simulink model "PowerSupplyTesting"  (R2022b)
settings: Solver=VariableStepAuto  StartTime=0.0  StopTime=10.0  RelTol=1e-3
libraries: fl_lib x60, ee_lib x28, batteryecm_lib x4
settings Model: Creator=minar  LastModifiedBy=minar

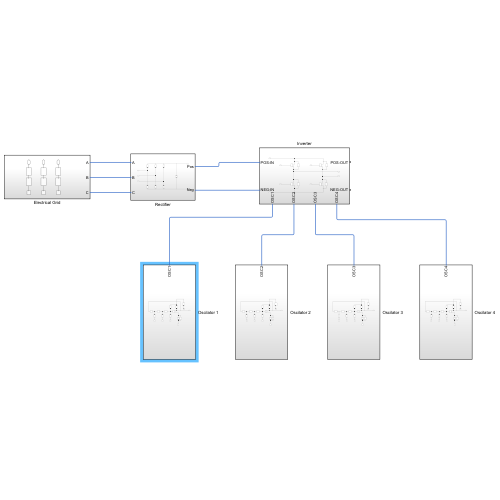
[thumbnail: Simulink's stored preview of the top-level diagram]
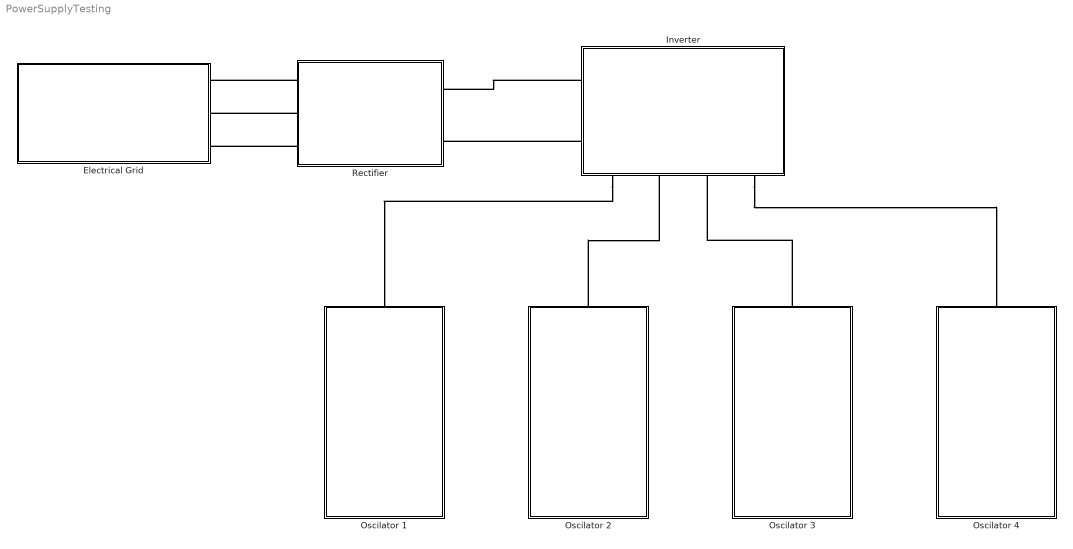
== system PowerSupplyTesting ==
  Electrical Grid : Subsystem
  Inverter : Subsystem
      settings: PortSchema="{\"entries\":[{\"content\":{\"sides\":[{\"content\":{\"connectorIds\":[\"LConn1\",\"LConn2\"]},\"type\":\"ConnectorPlacement.EquallySpacedRectSide\",\"uuid\":\"f7f5b9d2-2f28-4702-8197-1131bf06a0c8\"},{\"content\":{\"connectorIds\":[\"RConn1\",\"RConn2\"],\"side\":\"RIGHT\"},\"type\":\"ConnectorPlacement.EquallySpacedRectSide\",\"uuid\":\"68d9e126-9161-438e-ab0e-3e31da424ef3\"},{\"content\":{\"connectorIds\":[],\"side\":\"TOP\"},\"type\":\"ConnectorPlacement.EquallySpacedRectSide\",\"uuid\":\"a7ff2f77-40f7-4f33-b738-27e4211ddf2a\"},{\"content\":{\"connectorIds\":[\"RConn3\",\"RConn4\",\"RConn5\",\"RConn6\"],\"side\":\"BOTTOM\"},\"type\":\"ConnectorPlacement.EquallySpacedRectSide\",\"uuid\":\"8e7afd57-a60f-4a52-b345-b2d1ae69a6c4\"}]},\"type\":\"ConnectorPlacement.EquallySpacedConnector\",\"uuid\":\"2195a2bc-5e19-43d1-a283-5b386a715552\"}],\"packageUris\":[\"http://schema.mathworks.com/mf0/Connector/R2020b\"],\"version\":\"1.0\"}"
  Oscilator 1 : Subsystem
  Oscilator 2 : Subsystem
  Oscilator 3 : Subsystem
  Oscilator 4 : Subsystem
  Rectifier : Subsystem
  connections:
  Rectifier/RConn1 -- Electrical Grid/RConn1
  Rectifier/RConn2 -- Electrical Grid/RConn2
  Rectifier/RConn3 -- Electrical Grid/RConn3
  Inverter/LConn2 -- Rectifier/LConn2
  Inverter/LConn1 -- Rectifier/LConn1
  Oscilator 3/RConn1 -- Inverter/RConn5
  Oscilator 2/RConn1 -- Inverter/RConn4
  Inverter/RConn3 -- Oscilator 1/RConn1
  Inverter/RConn6 -- Oscilator 4/RConn1

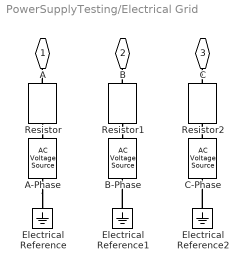
== system PowerSupplyTesting/Electrical Grid ==
  A-Phase : fl_lib/Electrical/Electrical Sources/AC Voltage Source  amp=208 V  shift=0 deg  frequency=60 Hz  omega=0 rad/s
  B-Phase : fl_lib/Electrical/Electrical Sources/AC Voltage Source  amp=208 V  shift=-120 deg  frequency=60 Hz  omega=0 rad/s
  C-Phase : fl_lib/Electrical/Electrical Sources/AC Voltage Source  amp=208 V  shift=-240 deg  frequency=60 Hz  omega=0 rad/s
  Electrical Reference : fl_lib/Electrical/Electrical Elements/Electrical Reference
  Electrical Reference1 : fl_lib/Electrical/Electrical Elements/Electrical Reference
  Electrical Reference2 : fl_lib/Electrical/Electrical Elements/Electrical Reference
  Resistor : fl_lib/Electrical/Electrical Elements/Resistor  R=0.1 Ohm  i_specify=off  i_priority=None  i=0 A  i_nominal_specify=off  i_nominal_unit=A  i_nominal_value=1  v_specify=off  v_priority=None  v=0 V  v_nominal_specify=off  v_nominal_unit=V  v_nominal_value=1
  Resistor1 : fl_lib/Electrical/Electrical Elements/Resistor  R=0.1 Ohm  i_specify=off  i_priority=None  i=0 A  i_nominal_specify=off  i_nominal_unit=A  i_nominal_value=1  v_specify=off  v_priority=None  v=0 V  v_nominal_specify=off  v_nominal_unit=V  v_nominal_value=1
  Resistor2 : fl_lib/Electrical/Electrical Elements/Resistor  R=0.1 Ohm  i_specify=off  i_priority=None  i=0 A  i_nominal_specify=off  i_nominal_unit=A  i_nominal_value=1  v_specify=off  v_priority=None  v=0 V  v_nominal_specify=off  v_nominal_unit=V  v_nominal_value=1
  A : PMIOPort  Side=Right
  B : PMIOPort  Port=2  Side=Right
  C : PMIOPort  Port=3  Side=Right
  connections:
  C-Phase/LConn1 -- Resistor2/RConn1
  A-Phase/RConn1 -- Electrical Reference/LConn1
  Electrical Reference1/LConn1 -- B-Phase/RConn1
  Electrical Reference2/LConn1 -- C-Phase/RConn1
  Resistor/LConn1 -- A/RConn1
  Resistor/RConn1 -- A-Phase/LConn1
  Resistor1/LConn1 -- B/RConn1
  Resistor1/RConn1 -- B-Phase/LConn1
  Resistor2/LConn1 -- C/RConn1

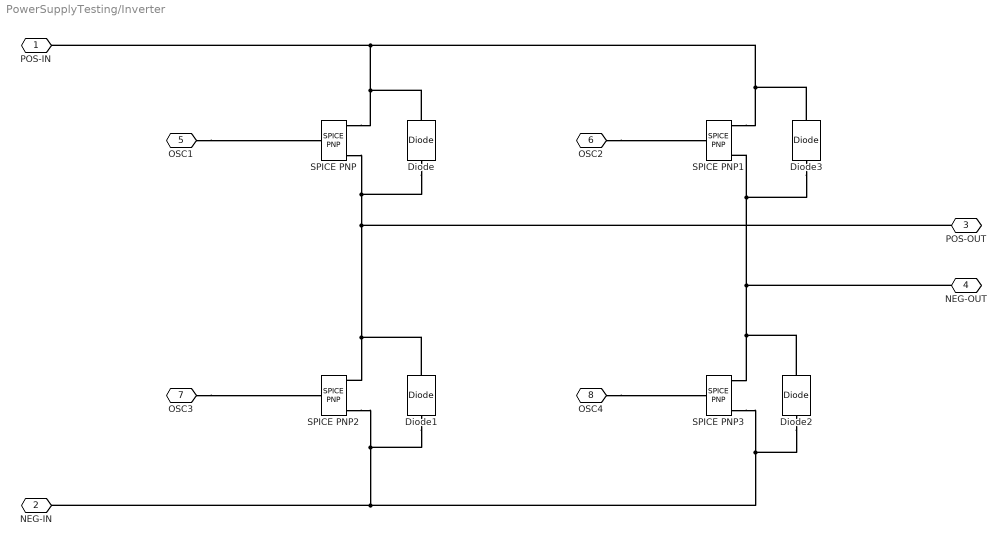
== system PowerSupplyTesting/Inverter ==
  Diode{,1..3} (4 alike) : ee_lib/Semiconductors & Converters/Diode  ModelType=ee.enum.diode.modelType.pwl  TableType=ee.enum.diode.tableType.IfMat  IfMat=[.07, .12, .19, 1.75, 4.24, 7.32, 11.2; .16, .3, .72, 2.14, 5.02, 8.35, 13.12] A  VfMat=[.9, 1.15, 1.25, 1.5, 1.75, 2.17, 2.6, 2.85; .58, .68, .75, 1.1, 1.38, 1.77, 2.27, 2.7] V  TjVec=[25, 125] degC  VfVec=[.5, .7, .9, 1.3, 1.7, 2.1, 2.5] V  IfVec=[.1, .2, .5, 1, 2, 4, 7, 10] A  Vf=0.6 V  Ron=0.3 Ohm  Goff=1e-8 S  prmExp=ee.enum.diode.expParam.useTwo  I12=[.0137, .545] A  V12=[.6, .7] V  RS=0 Ohm  Tmeas=25 degC  IS=1e-12 A  ec=1  I1=0.0137 A  V1=0.6 V  N_series=1  N_parallel=1  Rz=0.3 Ohm  BV=inf V  C_param=ee.enum.diode.capParam.fixed  CJ=0 pF  CJ0=5 pF  Vvec=[.1, 10, 100] V  Cvec=[3.5, 1, .4] pF  VJ=1 V  Mgrad=0.5  FC=0.5  Q_param=ee.enum.diode.recoveryParam.off  iRM=-7.15 A  iF=4 A  didt=-750 A/us  trr_factor=3  trr=115 ns  Qrr=150 nA*s  Vr=-600 V  Ls=150 nH  Erec=0.03 J  TT=50 ns  tau=100 ns  T_param=ee.enum.diode.temperatureParam.off  Tdevice=25 degC  I1_T2=0.245 A  V1_T2=0.5 V  IS_T2=1.25e-7 A  Tmeas2=125 degC  XTI_param=ee.enum.diode.xtiParam.pn  XTI=3  EG_param=ee.enum.diode.egapParam.material_si  EG=1.11 eV  dBVdT=0 V/K  enable_faults=simscape.enum.onoff.off  fault_action=simscape.enum.assert.action.none  fault_types=ee.enum.diode.faults.open  tau_fault=1e-3 s  IfMat_faulted=[.07, .12, .19, 1.75, 4.24, 7.32, 11.2; .16, .3, .72, 2.14, 4.02, 6.35, 9.12] A  VfMat_faulted=[.9, 1.15, 1.25, 1.5, 1.75, 2.17, 2.6, 2.85; .58, .68, .75, 1.1, 1.38, 1.77, 2.27, 2.7] V  VfVec_faulted=[.5, .7, .9, 1.3, 1.7, 2.1, 2.5] V  IfVec_faulted=[.1, .2, .5, 1, 2, 4, 7, 10] A  Ropen_faulted=1000 Ohm  Gshort_faulted=1000 1/Ohm  Vf_faulted=0.6 V  Ron_faulted=0.3 Ohm  Goff_faulted=1e-8 S  I12_faulted=[.0137, .545] A  V12_faulted=[.6, .7] V  IS_faulted=1e-12 A  ec_faulted=1  I1_faulted=0.0137 A  V1_faulted=0.6 V  RS_faulted=0 Ohm  Rz_faulted=0.3 Ohm  BV_faulted=inf V  Cscale_faulted=100  enable_temporal_fault=simscape.enum.onoff.off  t_fault=inf s  enable_behavioral_fault=simscape.enum.onoff.off  max_permissible_voltage=inf V  n_fail_on_voltage=1  max_permissible_current=inf A  t_fail_on_current=1 s  max_permissible_dVdt=inf V/s  enable_fault_input=simscape.enum.onoff.off  i_specify=off  i_priority=None  i=0 A  i_nominal_specify=off  i_nominal_unit=A  i_nominal_value=1  v_specify=off  v_priority=None  v=0 V  v_nominal_specify=off  v_nominal_unit=V  v_nominal_value=1  v_capacitor_specify=off  v_capacitor_priority=None  v_capacitor=0 V  v_capacitor_nominal_specify=off  v_capacitor_nominal_unit=V  v_capacitor_nominal_value=1  i_diode_specify=off  i_diode_priority=None  i_diode=0 A  i_diode_nominal_specify=off  i_diode_nominal_unit=A  i_diode_nominal_value=1  v_diode_specify=off  v_diode_priority=None  v_diode=0 V  v_diode_nominal_specify=off  v_diode_nominal_unit=V  v_diode_nominal_value=1  i_capacitor_specify=off  i_capacitor_priority=None  i_capacitor=0 A  i_capacitor_nominal_specify=off  i_capacitor_nominal_unit=A  i_capacitor_nominal_value=1  power_dissipated_specify=off  power_dissipated_priority=None  power_dissipated=0 W  power_dissipated_nominal_specify=off  power_dissipated_nominal_unit=W  power_dissipated_nominal_value=1  fidelity_level=ee.enum.diode.fidelity.includeChargeDyn  rec_loss_model=ee.enum.diode.reverseRecoveryModel.fixed  ErecVal=0 J  ErecMat=zeros(2, 3) J  TjrecVec=[298.15, 398.15] K  IfrecVec=[.1, 1, 10] A  VrecVal=10 V  tFilter=1 / 1000 / 100 s  max_permissible_temperature=inf K  t_fail_on_temperature=1 s  thermal_network_parameterization=ee.enum.thermalNetworkTopology.junctionCase  Rth=[0, 10] K/W  Rth_Cauer=[1, 3, 10] K/W  Rth_Foster=[4, 6] K/W  thermal_mass_parameterization=ee.enum.thermalNetwork.timeconstant  thermal_mass=[0, 1] J/K  thermal_mass_Cauer=[.1, .3, 1] J/K  thermal_mass_Foster=[1.5, 3] J/K  thermal_time_constant=[0, 10] s  thermal_time_constant_Cauer=[1, 3, 10] s  thermal_time_constant_Foster=[6, 18] s  thermal_mass_initial_temperatures=[25, 25] degC  thermal_mass_initial_temperatures_Cauer=[25, 25, 25] degC  junction_thermal_mass=0.01 J/K  Tvec_initial_Foster=[25, 25, 25, 25] degC  no_thermal_network=0  junction_temperature_specify=off  junction_temperature_priority=None  junction_temperature=25 degC  junction_temperature_nominal_specify=off  junction_temperature_nominal_unit=degC  junction_temperature_nominal_value=1
  SPICE PNP{,1..3} (4 alike) : ee_lib/Additional Components/SPICE Semiconductors/SPICE PNP  AREA=1.0 m^2  SCALE=1  IS=1.0e-16 A/m^2  BF=100.0  NF=1  VAF=Inf V  IKF=Inf A/m^2  ISE=0 A/m^2  NE=1.5  BR=1  NR=1  VAR=Inf V  IKR=Inf A/m^2  ISC=0 A/m^2  NC=2  RB=1 Ohm*m^2  IRB=Inf A/m^2  RBM=0 Ohm*m^2  RE=1e-4 Ohm*m^2  RC=0.01 Ohm*m^2  C_param=1  FC=0.5  IC_given=1  ICVBE=0 V  ICVCE=0 V  CJE=0 F/m^2  VJE=0.75 V  MJE=0.33  TF=0 s  XTF=0  VTF=Inf V  ITF=0 A/m^2  CJC=0 F/m^2  VJC=0.75 V  MJC=0.33  XCJC=1  TR=0 s  CJS=0 F/m^2  VJS=0.75 V  MJS=0  T_param=1  XTB=0  EG=1.11 eV  XTI=3  TFIXED=300.15 K  TMEAS=300.15 K  TOFFSET=0 K
      settings: InternalSimscapePortConfiguration="{\"Bottom\":[],\"Left\":[{\"id\":\"bx\",\"label\":\"\",\"type\":\"foundation.electrical.electrical\"}],\"Right\":[{\"id\":\"cx\",\"label\":\"\",\"type\":\"foundation.electrical.electrical\"},{\"id\":\"sx\",\"label\":\"s\",\"type\":\"foundation.electrical.electrical\"},{\"id\":\"ex\",\"label\":\"\",\"type\":\"foundation.electrical.electrical\"}],\"Top\":[]}"
  POS-IN : PMIOPort  Side=Left
  NEG-IN : PMIOPort  Port=2  Side=Left
  POS-OUT : PMIOPort  Port=3  Side=Right
  NEG-OUT : PMIOPort  Port=4  Side=Right
  OSC1 : PMIOPort  Port=5  Side=Right
  OSC2 : PMIOPort  Port=6  Side=Right
  OSC3 : PMIOPort  Port=7  Side=Right
  OSC4 : PMIOPort  Port=8  Side=Right
  connections:
  SPICE PNP3/RConn1 -- Diode2/LConn1 -- NEG-OUT/RConn1 -- Diode3/RConn1 -- SPICE PNP1/RConn3
  SPICE PNP/RConn3 -- Diode/RConn1 -- POS-OUT/RConn1 -- Diode1/LConn1 -- SPICE PNP2/RConn1
  OSC1/RConn1 -- SPICE PNP/LConn1
  OSC2/RConn1 -- SPICE PNP1/LConn1
  OSC3/RConn1 -- SPICE PNP2/LConn1
  OSC4/RConn1 -- SPICE PNP3/LConn1
  SPICE PNP2/RConn3 -- Diode1/RConn1 -- Diode2/RConn1 -- SPICE PNP3/RConn3 -- NEG-IN/RConn1
  SPICE PNP/RConn1 -- Diode/LConn1 -- Diode3/LConn1 -- SPICE PNP1/RConn1 -- POS-IN/RConn1

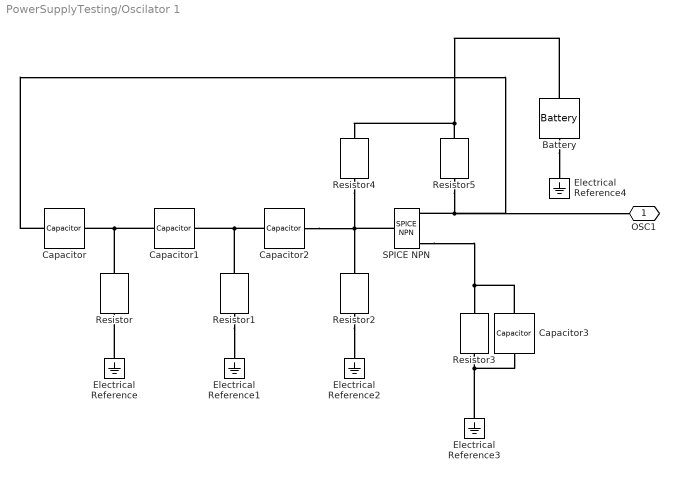
== system PowerSupplyTesting/Oscilator 1 ==
  Battery : batteryecm_lib/Battery  Vnom=12 V  prm_dir=simscape.enum.battery.prm_dir.disabled  R1_dis=2 Ohm  R1_ch=2 Ohm  R1=2 Ohm  prm_AH=simscape.enum.battery.prm_AH.infinite  AH=50 A*hr  V1=11.5 V  AH1=25 A*hr  prm_R2=simscape.enum.battery.prm_R2.disabled  R2=2000 Ohm  prm_dyn=simscape.enum.battery.prm_dyn.off  Rp1=0.005 Ohm  tau1=30 s  Rp2=0.005 Ohm  tau2=30 s  Rp3=0.005 Ohm  tau3=30 s  Rp4=0.005 Ohm  tau4=30 s  Rp5=0.005 Ohm  tau5=30 s  prm_fade=simscape.enum.battery.prm_fade.disabled  N_fade=100  AH_fade=45 A*hr  R1_fade=2.02 Ohm  R1_ch_fade=2.02 Ohm  V1_fade=10.35 V  prm_age=simscape.enum.battery.prm_age.disabled  prm_age_OCV=simscape.enum.battery.prm_age_OCV.OCV  OCV_age=0.9  SOC_age=60  delta_time_age_vec=[0] d  temperature_age_vec=[273] K  OCV_scaling_age=2.2134e6  OCV_offset_age=1.632e6  temp_exp_age=0.515833569 V  t_exp_age=0.75  i_specify=off  i_priority=None  i=0 A  i_nominal_specify=off  i_nominal_unit=A  i_nominal_value=1  v_specify=off  v_priority=None  v=0 V  v_nominal_specify=off  v_nominal_unit=V  v_nominal_value=1  charge_specify=off  charge_priority=High  charge=50 A*hr  charge_nominal_specify=off  charge_nominal_unit=A*hr  charge_nominal_value=1  num_cycles_specify=off  num_cycles_priority=High  num_cycles=0  num_cycles_nominal_specify=off  num_cycles_nominal_unit=1  num_cycles_nominal_value=1  Tmeas=298.15 K  Tmeas_age=298.15 K  Vnom_T2=12 V  R1_T2=2.2 Ohm  R1_T2_dis=2.2 Ohm  R1_T2_ch=2.2 Ohm  V1_T2=11.4 V  R2_T2=2200 Ohm  Rp1_T2=0.005 Ohm  tau1_T2=30 s  Rp2_T2=0.005 Ohm  tau2_T2=30 s  Rp3_T2=0.005 Ohm  tau3_T2=30 s  Rp4_T2=0.005 Ohm  tau4_T2=30 s  Rp5_T2=0.005 Ohm  tau5_T2=30 s  Tmeas2=273.15 K  thermal_mass=30000 J/K  temperature_specify=off  temperature_priority=High  temperature=298.15 K  temperature_nominal_specify=off  temperature_nominal_unit=K  temperature_nominal_value=1
  Capacitor{,1..3} (4 alike) : ee_lib/Passive/Capacitor  cap_option=0  c=1e-6 F  Cvec=[1e-05, 1e-06] F  Vvec=[0, 10] V  CV_table_symmetry=1  f_vec=[1, 10] kHz  DFext_vec=[.8, 1.2]  enable_C_tol=0  C_tol=5  tol_distribution=1  nSigma=4  r=1e-6 Ohm  g=0 1/Ohm  averaging_period=0 s  enable_operating_limits=0  operating_limit_action=2  max_working_voltage_range=[-25, 25] V  power_rating=1 W  enable_faults=0  fault_action=1  Cscale_faulted=100  R_faulted=1e-3 Ohm  G_faulted=0 1/Ohm  tau_fault=1e-3 s  enable_temporal_fault=0  t_fault=1 s  enable_behavioral_fault=0  max_permissible_voltage_range=[-100, 100] V  t_fail_on_voltage=1 s  i_specify=off  i_priority=None  i=0 A  i_nominal_specify=off  i_nominal_unit=A  i_nominal_value=1  v_specify=off  v_priority=None  v=0 V  v_nominal_specify=off  v_nominal_unit=V  v_nominal_value=1  vc_specify=off  vc_priority=High  vc=0 V  vc_nominal_specify=off  vc_nominal_unit=V  vc_nominal_value=1
  Electrical Reference{,1..4} (5 alike) : fl_lib/Electrical/Electrical Elements/Electrical Reference
  Resistor{,1..5} (6 alike) : fl_lib/Electrical/Electrical Elements/Resistor  R=1 Ohm  i_specify=off  i_priority=None  i=0 A  i_nominal_specify=off  i_nominal_unit=A  i_nominal_value=1  v_specify=off  v_priority=None  v=0 V  v_nominal_specify=off  v_nominal_unit=V  v_nominal_value=1
  SPICE NPN : ee_lib/Additional Components/SPICE Semiconductors/SPICE NPN  AREA=1.0 m^2  SCALE=1  IS=1.0e-16 A/m^2  BF=100.0  NF=1  VAF=Inf V  IKF=Inf A/m^2  ISE=0 A/m^2  NE=1.5  BR=1  NR=1  VAR=Inf V  IKR=Inf A/m^2  ISC=0 A/m^2  NC=2  RB=1 Ohm*m^2  IRB=Inf A/m^2  RBM=0 Ohm*m^2  RE=1e-4 Ohm*m^2  RC=0.01 Ohm*m^2  C_param=1  FC=0.5  IC_given=1  ICVBE=0 V  ICVCE=0 V  CJE=0 F/m^2  VJE=0.75 V  MJE=0.33  TF=0 s  XTF=0  VTF=Inf V  ITF=0 A/m^2  CJC=0 F/m^2  VJC=0.75 V  MJC=0.33  XCJC=1  TR=0 s  CJS=0 F/m^2  VJS=0.75 V  MJS=0  T_param=1  XTB=0  EG=1.11 eV  XTI=3  TFIXED=300.15 K  TMEAS=300.15 K  TOFFSET=0 K
      settings: InternalSimscapePortConfiguration="{\"Bottom\":[],\"Left\":[{\"id\":\"bx\",\"label\":\"\",\"type\":\"foundation.electrical.electrical\"}],\"Right\":[{\"id\":\"cx\",\"label\":\"\",\"type\":\"foundation.electrical.electrical\"},{\"id\":\"sx\",\"label\":\"s\",\"type\":\"foundation.electrical.electrical\"},{\"id\":\"ex\",\"label\":\"\",\"type\":\"foundation.electrical.electrical\"}],\"Top\":[]}"
  OSC1 : PMIOPort  Side=Right
  connections:
  SPICE NPN/RConn3 -- Capacitor3/LConn1 -- Resistor3/LConn1
  Capacitor3/RConn1 -- Electrical Reference3/LConn1 -- Resistor3/RConn1
  Resistor5/RConn1 -- OSC1/RConn1 -- Capacitor/LConn1 -- SPICE NPN/RConn1
  Resistor5/LConn1 -- Battery/LConn1 -- Resistor4/LConn1
  Resistor4/RConn1 -- Resistor2/LConn1 -- Capacitor2/RConn1 -- SPICE NPN/LConn1
  Capacitor2/LConn1 -- Capacitor1/RConn1 -- Resistor1/LConn1
  Capacitor1/LConn1 -- Resistor/LConn1 -- Capacitor/RConn1
  Electrical Reference/LConn1 -- Resistor/RConn1
  Resistor1/RConn1 -- Electrical Reference1/LConn1
  Resistor2/RConn1 -- Electrical Reference2/LConn1
  Battery/RConn1 -- Electrical Reference4/LConn1

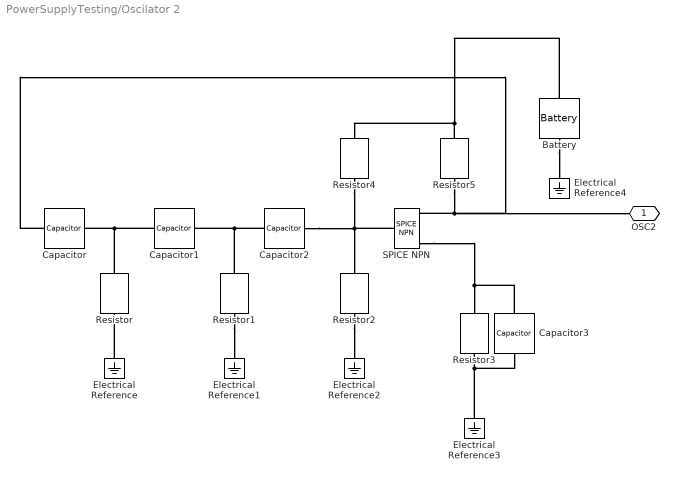
== system PowerSupplyTesting/Oscilator 2 ==
  Battery : batteryecm_lib/Battery  Vnom=12 V  prm_dir=simscape.enum.battery.prm_dir.disabled  R1_dis=2 Ohm  R1_ch=2 Ohm  R1=2 Ohm  prm_AH=simscape.enum.battery.prm_AH.infinite  AH=50 A*hr  V1=11.5 V  AH1=25 A*hr  prm_R2=simscape.enum.battery.prm_R2.disabled  R2=2000 Ohm  prm_dyn=simscape.enum.battery.prm_dyn.off  Rp1=0.005 Ohm  tau1=30 s  Rp2=0.005 Ohm  tau2=30 s  Rp3=0.005 Ohm  tau3=30 s  Rp4=0.005 Ohm  tau4=30 s  Rp5=0.005 Ohm  tau5=30 s  prm_fade=simscape.enum.battery.prm_fade.disabled  N_fade=100  AH_fade=45 A*hr  R1_fade=2.02 Ohm  R1_ch_fade=2.02 Ohm  V1_fade=10.35 V  prm_age=simscape.enum.battery.prm_age.disabled  prm_age_OCV=simscape.enum.battery.prm_age_OCV.OCV  OCV_age=0.9  SOC_age=60  delta_time_age_vec=[0] d  temperature_age_vec=[273] K  OCV_scaling_age=2.2134e6  OCV_offset_age=1.632e6  temp_exp_age=0.515833569 V  t_exp_age=0.75  i_specify=off  i_priority=None  i=0 A  i_nominal_specify=off  i_nominal_unit=A  i_nominal_value=1  v_specify=off  v_priority=None  v=0 V  v_nominal_specify=off  v_nominal_unit=V  v_nominal_value=1  charge_specify=off  charge_priority=High  charge=50 A*hr  charge_nominal_specify=off  charge_nominal_unit=A*hr  charge_nominal_value=1  num_cycles_specify=off  num_cycles_priority=High  num_cycles=0  num_cycles_nominal_specify=off  num_cycles_nominal_unit=1  num_cycles_nominal_value=1  Tmeas=298.15 K  Tmeas_age=298.15 K  Vnom_T2=12 V  R1_T2=2.2 Ohm  R1_T2_dis=2.2 Ohm  R1_T2_ch=2.2 Ohm  V1_T2=11.4 V  R2_T2=2200 Ohm  Rp1_T2=0.005 Ohm  tau1_T2=30 s  Rp2_T2=0.005 Ohm  tau2_T2=30 s  Rp3_T2=0.005 Ohm  tau3_T2=30 s  Rp4_T2=0.005 Ohm  tau4_T2=30 s  Rp5_T2=0.005 Ohm  tau5_T2=30 s  Tmeas2=273.15 K  thermal_mass=30000 J/K  temperature_specify=off  temperature_priority=High  temperature=298.15 K  temperature_nominal_specify=off  temperature_nominal_unit=K  temperature_nominal_value=1
  Capacitor{,1..3} (4 alike) : ee_lib/Passive/Capacitor  cap_option=0  c=1e-6 F  Cvec=[1e-05, 1e-06] F  Vvec=[0, 10] V  CV_table_symmetry=1  f_vec=[1, 10] kHz  DFext_vec=[.8, 1.2]  enable_C_tol=0  C_tol=5  tol_distribution=1  nSigma=4  r=1e-6 Ohm  g=0 1/Ohm  averaging_period=0 s  enable_operating_limits=0  operating_limit_action=2  max_working_voltage_range=[-25, 25] V  power_rating=1 W  enable_faults=0  fault_action=1  Cscale_faulted=100  R_faulted=1e-3 Ohm  G_faulted=0 1/Ohm  tau_fault=1e-3 s  enable_temporal_fault=0  t_fault=1 s  enable_behavioral_fault=0  max_permissible_voltage_range=[-100, 100] V  t_fail_on_voltage=1 s  i_specify=off  i_priority=None  i=0 A  i_nominal_specify=off  i_nominal_unit=A  i_nominal_value=1  v_specify=off  v_priority=None  v=0 V  v_nominal_specify=off  v_nominal_unit=V  v_nominal_value=1  vc_specify=off  vc_priority=High  vc=0 V  vc_nominal_specify=off  vc_nominal_unit=V  vc_nominal_value=1
  Electrical Reference{,1..4} (5 alike) : fl_lib/Electrical/Electrical Elements/Electrical Reference
  Resistor{,1..5} (6 alike) : fl_lib/Electrical/Electrical Elements/Resistor  R=1 Ohm  i_specify=off  i_priority=None  i=0 A  i_nominal_specify=off  i_nominal_unit=A  i_nominal_value=1  v_specify=off  v_priority=None  v=0 V  v_nominal_specify=off  v_nominal_unit=V  v_nominal_value=1
  SPICE NPN : ee_lib/Additional Components/SPICE Semiconductors/SPICE NPN  AREA=1.0 m^2  SCALE=1  IS=1.0e-16 A/m^2  BF=100.0  NF=1  VAF=Inf V  IKF=Inf A/m^2  ISE=0 A/m^2  NE=1.5  BR=1  NR=1  VAR=Inf V  IKR=Inf A/m^2  ISC=0 A/m^2  NC=2  RB=1 Ohm*m^2  IRB=Inf A/m^2  RBM=0 Ohm*m^2  RE=1e-4 Ohm*m^2  RC=0.01 Ohm*m^2  C_param=1  FC=0.5  IC_given=1  ICVBE=0 V  ICVCE=0 V  CJE=0 F/m^2  VJE=0.75 V  MJE=0.33  TF=0 s  XTF=0  VTF=Inf V  ITF=0 A/m^2  CJC=0 F/m^2  VJC=0.75 V  MJC=0.33  XCJC=1  TR=0 s  CJS=0 F/m^2  VJS=0.75 V  MJS=0  T_param=1  XTB=0  EG=1.11 eV  XTI=3  TFIXED=300.15 K  TMEAS=300.15 K  TOFFSET=0 K
      settings: InternalSimscapePortConfiguration="{\"Bottom\":[],\"Left\":[{\"id\":\"bx\",\"label\":\"\",\"type\":\"foundation.electrical.electrical\"}],\"Right\":[{\"id\":\"cx\",\"label\":\"\",\"type\":\"foundation.electrical.electrical\"},{\"id\":\"sx\",\"label\":\"s\",\"type\":\"foundation.electrical.electrical\"},{\"id\":\"ex\",\"label\":\"\",\"type\":\"foundation.electrical.electrical\"}],\"Top\":[]}"
  OSC2 : PMIOPort  Side=Right
  connections:
  SPICE NPN/RConn3 -- Capacitor3/LConn1 -- Resistor3/LConn1
  Capacitor3/RConn1 -- Electrical Reference3/LConn1 -- Resistor3/RConn1
  Resistor5/RConn1 -- OSC2/RConn1 -- Capacitor/LConn1 -- SPICE NPN/RConn1
  Resistor5/LConn1 -- Battery/LConn1 -- Resistor4/LConn1
  Resistor4/RConn1 -- Resistor2/LConn1 -- Capacitor2/RConn1 -- SPICE NPN/LConn1
  Capacitor2/LConn1 -- Capacitor1/RConn1 -- Resistor1/LConn1
  Capacitor1/LConn1 -- Resistor/LConn1 -- Capacitor/RConn1
  Electrical Reference/LConn1 -- Resistor/RConn1
  Resistor1/RConn1 -- Electrical Reference1/LConn1
  Resistor2/RConn1 -- Electrical Reference2/LConn1
  Battery/RConn1 -- Electrical Reference4/LConn1

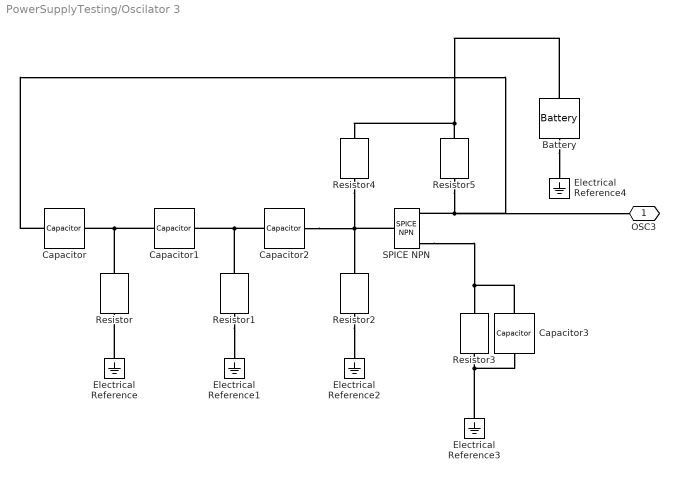
== system PowerSupplyTesting/Oscilator 3 ==
  Battery : batteryecm_lib/Battery  Vnom=12 V  prm_dir=simscape.enum.battery.prm_dir.disabled  R1_dis=2 Ohm  R1_ch=2 Ohm  R1=2 Ohm  prm_AH=simscape.enum.battery.prm_AH.infinite  AH=50 A*hr  V1=11.5 V  AH1=25 A*hr  prm_R2=simscape.enum.battery.prm_R2.disabled  R2=2000 Ohm  prm_dyn=simscape.enum.battery.prm_dyn.off  Rp1=0.005 Ohm  tau1=30 s  Rp2=0.005 Ohm  tau2=30 s  Rp3=0.005 Ohm  tau3=30 s  Rp4=0.005 Ohm  tau4=30 s  Rp5=0.005 Ohm  tau5=30 s  prm_fade=simscape.enum.battery.prm_fade.disabled  N_fade=100  AH_fade=45 A*hr  R1_fade=2.02 Ohm  R1_ch_fade=2.02 Ohm  V1_fade=10.35 V  prm_age=simscape.enum.battery.prm_age.disabled  prm_age_OCV=simscape.enum.battery.prm_age_OCV.OCV  OCV_age=0.9  SOC_age=60  delta_time_age_vec=[0] d  temperature_age_vec=[273] K  OCV_scaling_age=2.2134e6  OCV_offset_age=1.632e6  temp_exp_age=0.515833569 V  t_exp_age=0.75  i_specify=off  i_priority=None  i=0 A  i_nominal_specify=off  i_nominal_unit=A  i_nominal_value=1  v_specify=off  v_priority=None  v=0 V  v_nominal_specify=off  v_nominal_unit=V  v_nominal_value=1  charge_specify=off  charge_priority=High  charge=50 A*hr  charge_nominal_specify=off  charge_nominal_unit=A*hr  charge_nominal_value=1  num_cycles_specify=off  num_cycles_priority=High  num_cycles=0  num_cycles_nominal_specify=off  num_cycles_nominal_unit=1  num_cycles_nominal_value=1  Tmeas=298.15 K  Tmeas_age=298.15 K  Vnom_T2=12 V  R1_T2=2.2 Ohm  R1_T2_dis=2.2 Ohm  R1_T2_ch=2.2 Ohm  V1_T2=11.4 V  R2_T2=2200 Ohm  Rp1_T2=0.005 Ohm  tau1_T2=30 s  Rp2_T2=0.005 Ohm  tau2_T2=30 s  Rp3_T2=0.005 Ohm  tau3_T2=30 s  Rp4_T2=0.005 Ohm  tau4_T2=30 s  Rp5_T2=0.005 Ohm  tau5_T2=30 s  Tmeas2=273.15 K  thermal_mass=30000 J/K  temperature_specify=off  temperature_priority=High  temperature=298.15 K  temperature_nominal_specify=off  temperature_nominal_unit=K  temperature_nominal_value=1
  Capacitor{,1..3} (4 alike) : ee_lib/Passive/Capacitor  cap_option=0  c=1e-6 F  Cvec=[1e-05, 1e-06] F  Vvec=[0, 10] V  CV_table_symmetry=1  f_vec=[1, 10] kHz  DFext_vec=[.8, 1.2]  enable_C_tol=0  C_tol=5  tol_distribution=1  nSigma=4  r=1e-6 Ohm  g=0 1/Ohm  averaging_period=0 s  enable_operating_limits=0  operating_limit_action=2  max_working_voltage_range=[-25, 25] V  power_rating=1 W  enable_faults=0  fault_action=1  Cscale_faulted=100  R_faulted=1e-3 Ohm  G_faulted=0 1/Ohm  tau_fault=1e-3 s  enable_temporal_fault=0  t_fault=1 s  enable_behavioral_fault=0  max_permissible_voltage_range=[-100, 100] V  t_fail_on_voltage=1 s  i_specify=off  i_priority=None  i=0 A  i_nominal_specify=off  i_nominal_unit=A  i_nominal_value=1  v_specify=off  v_priority=None  v=0 V  v_nominal_specify=off  v_nominal_unit=V  v_nominal_value=1  vc_specify=off  vc_priority=High  vc=0 V  vc_nominal_specify=off  vc_nominal_unit=V  vc_nominal_value=1
  Electrical Reference{,1..4} (5 alike) : fl_lib/Electrical/Electrical Elements/Electrical Reference
  Resistor{,1..5} (6 alike) : fl_lib/Electrical/Electrical Elements/Resistor  R=1 Ohm  i_specify=off  i_priority=None  i=0 A  i_nominal_specify=off  i_nominal_unit=A  i_nominal_value=1  v_specify=off  v_priority=None  v=0 V  v_nominal_specify=off  v_nominal_unit=V  v_nominal_value=1
  SPICE NPN : ee_lib/Additional Components/SPICE Semiconductors/SPICE NPN  AREA=1.0 m^2  SCALE=1  IS=1.0e-16 A/m^2  BF=100.0  NF=1  VAF=Inf V  IKF=Inf A/m^2  ISE=0 A/m^2  NE=1.5  BR=1  NR=1  VAR=Inf V  IKR=Inf A/m^2  ISC=0 A/m^2  NC=2  RB=1 Ohm*m^2  IRB=Inf A/m^2  RBM=0 Ohm*m^2  RE=1e-4 Ohm*m^2  RC=0.01 Ohm*m^2  C_param=1  FC=0.5  IC_given=1  ICVBE=0 V  ICVCE=0 V  CJE=0 F/m^2  VJE=0.75 V  MJE=0.33  TF=0 s  XTF=0  VTF=Inf V  ITF=0 A/m^2  CJC=0 F/m^2  VJC=0.75 V  MJC=0.33  XCJC=1  TR=0 s  CJS=0 F/m^2  VJS=0.75 V  MJS=0  T_param=1  XTB=0  EG=1.11 eV  XTI=3  TFIXED=300.15 K  TMEAS=300.15 K  TOFFSET=0 K
      settings: InternalSimscapePortConfiguration="{\"Bottom\":[],\"Left\":[{\"id\":\"bx\",\"label\":\"\",\"type\":\"foundation.electrical.electrical\"}],\"Right\":[{\"id\":\"cx\",\"label\":\"\",\"type\":\"foundation.electrical.electrical\"},{\"id\":\"sx\",\"label\":\"s\",\"type\":\"foundation.electrical.electrical\"},{\"id\":\"ex\",\"label\":\"\",\"type\":\"foundation.electrical.electrical\"}],\"Top\":[]}"
  OSC3 : PMIOPort  Side=Right
  connections:
  SPICE NPN/RConn3 -- Capacitor3/LConn1 -- Resistor3/LConn1
  Capacitor3/RConn1 -- Electrical Reference3/LConn1 -- Resistor3/RConn1
  Resistor5/RConn1 -- OSC3/RConn1 -- Capacitor/LConn1 -- SPICE NPN/RConn1
  Resistor5/LConn1 -- Battery/LConn1 -- Resistor4/LConn1
  Resistor4/RConn1 -- Resistor2/LConn1 -- Capacitor2/RConn1 -- SPICE NPN/LConn1
  Capacitor2/LConn1 -- Capacitor1/RConn1 -- Resistor1/LConn1
  Capacitor1/LConn1 -- Resistor/LConn1 -- Capacitor/RConn1
  Electrical Reference/LConn1 -- Resistor/RConn1
  Resistor1/RConn1 -- Electrical Reference1/LConn1
  Resistor2/RConn1 -- Electrical Reference2/LConn1
  Battery/RConn1 -- Electrical Reference4/LConn1

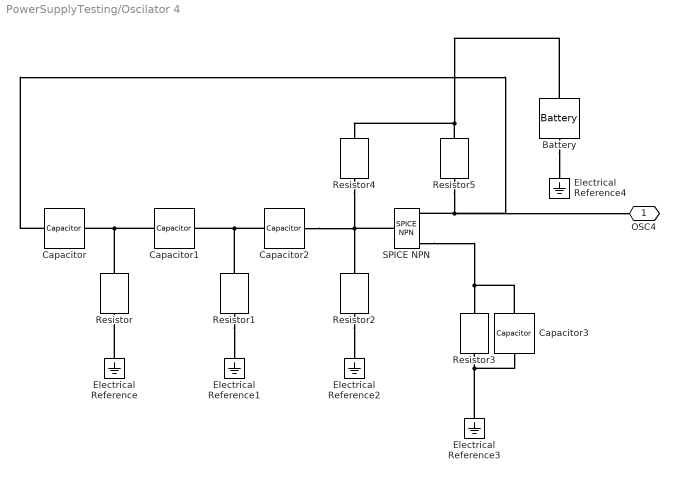
== system PowerSupplyTesting/Oscilator 4 ==
  Battery : batteryecm_lib/Battery  Vnom=12 V  prm_dir=simscape.enum.battery.prm_dir.disabled  R1_dis=2 Ohm  R1_ch=2 Ohm  R1=2 Ohm  prm_AH=simscape.enum.battery.prm_AH.infinite  AH=50 A*hr  V1=11.5 V  AH1=25 A*hr  prm_R2=simscape.enum.battery.prm_R2.disabled  R2=2000 Ohm  prm_dyn=simscape.enum.battery.prm_dyn.off  Rp1=0.005 Ohm  tau1=30 s  Rp2=0.005 Ohm  tau2=30 s  Rp3=0.005 Ohm  tau3=30 s  Rp4=0.005 Ohm  tau4=30 s  Rp5=0.005 Ohm  tau5=30 s  prm_fade=simscape.enum.battery.prm_fade.disabled  N_fade=100  AH_fade=45 A*hr  R1_fade=2.02 Ohm  R1_ch_fade=2.02 Ohm  V1_fade=10.35 V  prm_age=simscape.enum.battery.prm_age.disabled  prm_age_OCV=simscape.enum.battery.prm_age_OCV.OCV  OCV_age=0.9  SOC_age=60  delta_time_age_vec=[0] d  temperature_age_vec=[273] K  OCV_scaling_age=2.2134e6  OCV_offset_age=1.632e6  temp_exp_age=0.515833569 V  t_exp_age=0.75  i_specify=off  i_priority=None  i=0 A  i_nominal_specify=off  i_nominal_unit=A  i_nominal_value=1  v_specify=off  v_priority=None  v=0 V  v_nominal_specify=off  v_nominal_unit=V  v_nominal_value=1  charge_specify=off  charge_priority=High  charge=50 A*hr  charge_nominal_specify=off  charge_nominal_unit=A*hr  charge_nominal_value=1  num_cycles_specify=off  num_cycles_priority=High  num_cycles=0  num_cycles_nominal_specify=off  num_cycles_nominal_unit=1  num_cycles_nominal_value=1  Tmeas=298.15 K  Tmeas_age=298.15 K  Vnom_T2=12 V  R1_T2=2.2 Ohm  R1_T2_dis=2.2 Ohm  R1_T2_ch=2.2 Ohm  V1_T2=11.4 V  R2_T2=2200 Ohm  Rp1_T2=0.005 Ohm  tau1_T2=30 s  Rp2_T2=0.005 Ohm  tau2_T2=30 s  Rp3_T2=0.005 Ohm  tau3_T2=30 s  Rp4_T2=0.005 Ohm  tau4_T2=30 s  Rp5_T2=0.005 Ohm  tau5_T2=30 s  Tmeas2=273.15 K  thermal_mass=30000 J/K  temperature_specify=off  temperature_priority=High  temperature=298.15 K  temperature_nominal_specify=off  temperature_nominal_unit=K  temperature_nominal_value=1
  Capacitor{,1..3} (4 alike) : ee_lib/Passive/Capacitor  cap_option=0  c=1e-6 F  Cvec=[1e-05, 1e-06] F  Vvec=[0, 10] V  CV_table_symmetry=1  f_vec=[1, 10] kHz  DFext_vec=[.8, 1.2]  enable_C_tol=0  C_tol=5  tol_distribution=1  nSigma=4  r=1e-6 Ohm  g=0 1/Ohm  averaging_period=0 s  enable_operating_limits=0  operating_limit_action=2  max_working_voltage_range=[-25, 25] V  power_rating=1 W  enable_faults=0  fault_action=1  Cscale_faulted=100  R_faulted=1e-3 Ohm  G_faulted=0 1/Ohm  tau_fault=1e-3 s  enable_temporal_fault=0  t_fault=1 s  enable_behavioral_fault=0  max_permissible_voltage_range=[-100, 100] V  t_fail_on_voltage=1 s  i_specify=off  i_priority=None  i=0 A  i_nominal_specify=off  i_nominal_unit=A  i_nominal_value=1  v_specify=off  v_priority=None  v=0 V  v_nominal_specify=off  v_nominal_unit=V  v_nominal_value=1  vc_specify=off  vc_priority=High  vc=0 V  vc_nominal_specify=off  vc_nominal_unit=V  vc_nominal_value=1
  Electrical Reference{,1..4} (5 alike) : fl_lib/Electrical/Electrical Elements/Electrical Reference
  Resistor{,1..5} (6 alike) : fl_lib/Electrical/Electrical Elements/Resistor  R=1 Ohm  i_specify=off  i_priority=None  i=0 A  i_nominal_specify=off  i_nominal_unit=A  i_nominal_value=1  v_specify=off  v_priority=None  v=0 V  v_nominal_specify=off  v_nominal_unit=V  v_nominal_value=1
  SPICE NPN : ee_lib/Additional Components/SPICE Semiconductors/SPICE NPN  AREA=1.0 m^2  SCALE=1  IS=1.0e-16 A/m^2  BF=100.0  NF=1  VAF=Inf V  IKF=Inf A/m^2  ISE=0 A/m^2  NE=1.5  BR=1  NR=1  VAR=Inf V  IKR=Inf A/m^2  ISC=0 A/m^2  NC=2  RB=1 Ohm*m^2  IRB=Inf A/m^2  RBM=0 Ohm*m^2  RE=1e-4 Ohm*m^2  RC=0.01 Ohm*m^2  C_param=1  FC=0.5  IC_given=1  ICVBE=0 V  ICVCE=0 V  CJE=0 F/m^2  VJE=0.75 V  MJE=0.33  TF=0 s  XTF=0  VTF=Inf V  ITF=0 A/m^2  CJC=0 F/m^2  VJC=0.75 V  MJC=0.33  XCJC=1  TR=0 s  CJS=0 F/m^2  VJS=0.75 V  MJS=0  T_param=1  XTB=0  EG=1.11 eV  XTI=3  TFIXED=300.15 K  TMEAS=300.15 K  TOFFSET=0 K
      settings: InternalSimscapePortConfiguration="{\"Bottom\":[],\"Left\":[{\"id\":\"bx\",\"label\":\"\",\"type\":\"foundation.electrical.electrical\"}],\"Right\":[{\"id\":\"cx\",\"label\":\"\",\"type\":\"foundation.electrical.electrical\"},{\"id\":\"sx\",\"label\":\"s\",\"type\":\"foundation.electrical.electrical\"},{\"id\":\"ex\",\"label\":\"\",\"type\":\"foundation.electrical.electrical\"}],\"Top\":[]}"
  OSC4 : PMIOPort  Side=Right
  connections:
  SPICE NPN/RConn3 -- Capacitor3/LConn1 -- Resistor3/LConn1
  Capacitor3/RConn1 -- Electrical Reference3/LConn1 -- Resistor3/RConn1
  Resistor5/RConn1 -- OSC4/RConn1 -- Capacitor/LConn1 -- SPICE NPN/RConn1
  Resistor5/LConn1 -- Battery/LConn1 -- Resistor4/LConn1
  Resistor4/RConn1 -- Resistor2/LConn1 -- Capacitor2/RConn1 -- SPICE NPN/LConn1
  Capacitor2/LConn1 -- Capacitor1/RConn1 -- Resistor1/LConn1
  Capacitor1/LConn1 -- Resistor/LConn1 -- Capacitor/RConn1
  Electrical Reference/LConn1 -- Resistor/RConn1
  Resistor1/RConn1 -- Electrical Reference1/LConn1
  Resistor2/RConn1 -- Electrical Reference2/LConn1
  Battery/RConn1 -- Electrical Reference4/LConn1

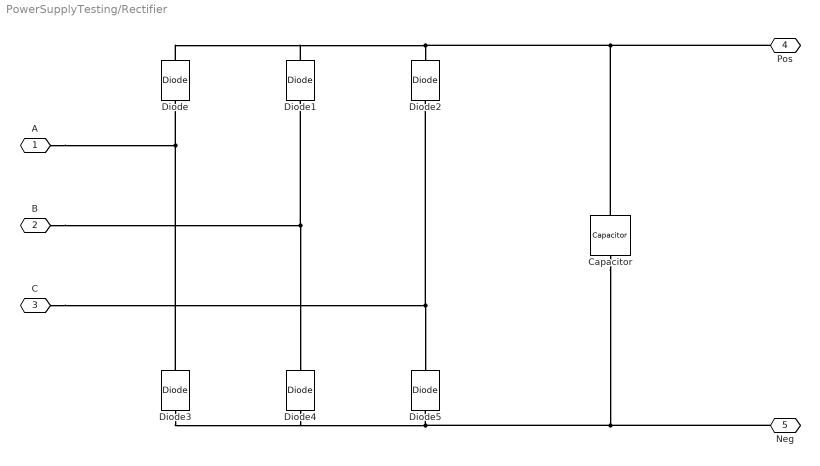
== system PowerSupplyTesting/Rectifier ==
  Capacitor : fl_lib/Electrical/Electrical Elements/Capacitor  c=1e-6 F  r=1e-6 Ohm  g=0 1/Ohm  i_specify=off  i_priority=None  i=0 A  i_nominal_specify=off  i_nominal_unit=A  i_nominal_value=1  v_specify=off  v_priority=None  v=0 V  v_nominal_specify=off  v_nominal_unit=V  v_nominal_value=1  vc_specify=off  vc_priority=High  vc=0 V  vc_nominal_specify=off  vc_nominal_unit=V  vc_nominal_value=1
  Diode{,1..5} (6 alike) : fl_lib/Electrical/Electrical Elements/Diode  Vf=0.6 V  Ron=0.3 Ohm  Goff=1e-8 1/Ohm  i_specify=off  i_priority=None  i=0 A  i_nominal_specify=off  i_nominal_unit=A  i_nominal_value=1  v_specify=off  v_priority=None  v=0 V  v_nominal_specify=off  v_nominal_unit=V  v_nominal_value=1
  A : PMIOPort  Side=Right
  B : PMIOPort  Port=2  Side=Right
  C : PMIOPort  Port=3  Side=Right
  Pos : PMIOPort  Port=4  Side=Left
  Neg : PMIOPort  Port=5  Side=Left
  connections:
  A/RConn1 -- Diode3/RConn1 -- Diode/LConn1
  B/RConn1 -- Diode4/RConn1 -- Diode1/LConn1
  C/RConn1 -- Diode5/RConn1 -- Diode2/LConn1
  Capacitor/LConn1 -- Pos/RConn1 -- Diode/RConn1 -- Diode1/RConn1 -- Diode2/RConn1
  Capacitor/RConn1 -- Neg/RConn1 -- Diode3/LConn1 -- Diode4/LConn1 -- Diode5/LConn1
